simulink model "LAB4_Quanser"  (R2021b)
settings: Solver=VariableStepAuto  StartTime=0.0  StopTime=100  FixedStep=Ts  RelTol=1e-3
InitFcn:
  | Ts=1e-3;
  | Ra = 2.6+2;
  | Ka = 1/Ra;
  | Ta = 500e-6;
  | Tfi = 1e-3;
  | Tsum = 2e-3;
  | KR =1/(2*Ka)*Tfi/Tsum;
  | P = KR;
  | I = KR/Ta;
  | Tfb = 10e-3;
undefined symbols (not defined in the file): Model_626, Sensoray
libraries: sldrtlib x3, simulink x1
settings Model: SimulationMode=external  ExtModeTrigDuration=10001  Creator=Melab1Guest  LastModifiedBy=Marko
settings SolverCC: AlgebraicLoopSolver=TrustRegion
settings SFSimCC: CustomCodeUndefinedFunction=UseInterfaceOnly
settings RTWCC: Description=Simulink Desktop Real-Time  SystemTargetFile=sldrt.tlc  TemplateMakefile=sldrt.tmf  RTWCompilerOptimization=on
settings CodeAppCC: MaxIdLength=95
settings SimulinkDesktopRealTimeCC: TargetPreCompLibLocation=C:\Program Files\MATLAB\R2021b\toolbox\sldrt\lib\win64

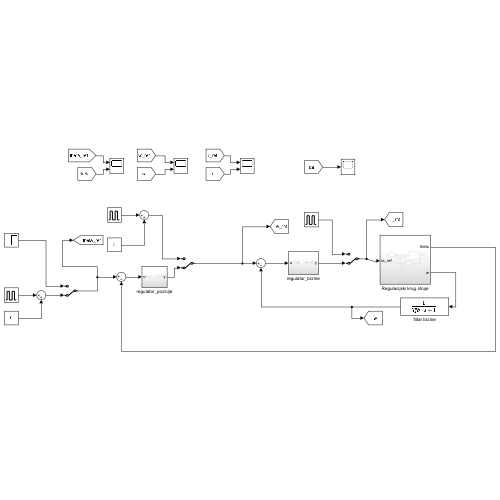
[thumbnail: Simulink's stored preview of the top-level diagram]
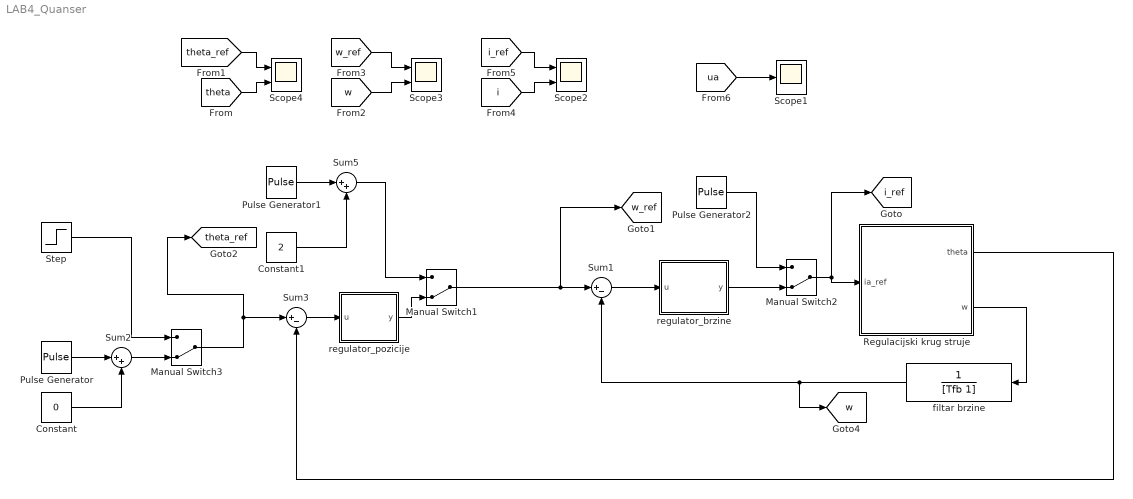
== system LAB4_Quanser ==
  Constant : Constant  Value=0
  Constant1 : Constant  Value=2
  Manual Switch1 : ManualSwitch  CurrentSetting=0
  Manual Switch2 : ManualSwitch  CurrentSetting=0
  Manual Switch3 : ManualSwitch  CurrentSetting=0
  Pulse Generator : DiscretePulseGenerator  PulseType=Time based  Period=10  PulseWidth=50
  Pulse Generator1 : DiscretePulseGenerator  PulseType=Time based  Period=5  PulseWidth=50
  Pulse Generator2 : DiscretePulseGenerator  PulseType=Time based  Amplitude=0.2  Period=3  PulseWidth=50
  Regulacijski krug struje : Subsystem
  Scope1 : Scope
  Scope2 : Scope  NumInputPorts=2
  Scope3 : Scope  NumInputPorts=2
  Scope4 : Scope  NumInputPorts=2
  Step : Step  SampleTime=0
  Sum1 : Sum  Inputs=|+-
  Sum2 : Sum  Inputs=|++
  Sum3 : Sum  Inputs=|+-
  Sum5 : Sum  Inputs=|++
  filtar brzine : TransferFcn  Denominator=[Tfb 1]
  regulator_brzine : Subsystem
  regulator_pozicije : Subsystem
  tag scope: i_ref=global, theta_ref=global, w=global, w_ref=global
  wires:
  Pulse Generator/1 -> Sum2/1
  Constant/1 -> Sum2/2
  Pulse Generator1/1 -> Sum5/1
  Constant1/1 -> Sum5/2
  Sum5/1 -> Manual Switch1/1
  Regulacijski krug struje/1(theta) -> Sum3/2
  Regulacijski krug struje/2(w) -> filtar brzine/1
  Manual Switch2/1 -> [i_ref], Regulacijski krug struje/1(ia_ref)
  Manual Switch3/1 -> Sum3/1, [theta_ref]
  Sum2/1 -> Manual Switch3/2
  Step/1 -> Manual Switch3/1
  filtar brzine/1 -> [w], Sum1/2
  [w_ref] -> Scope3/1
  [w] -> Scope3/2
  [theta] -> Scope4/2
  [theta_ref] -> Scope4/1
  [i_ref] -> Scope2/1
  [i] -> Scope2/2
  Sum3/1 -> regulator_pozicije/1(u)
  regulator_pozicije/1(y) -> Manual Switch1/2
  Sum1/1 -> regulator_brzine/1(u)
  regulator_brzine/1(y) -> Manual Switch2/2
  Pulse Generator2/1 -> Manual Switch2/1
  [ua] -> Scope1/1
  Manual Switch1/1 -> [w_ref], Sum1/1

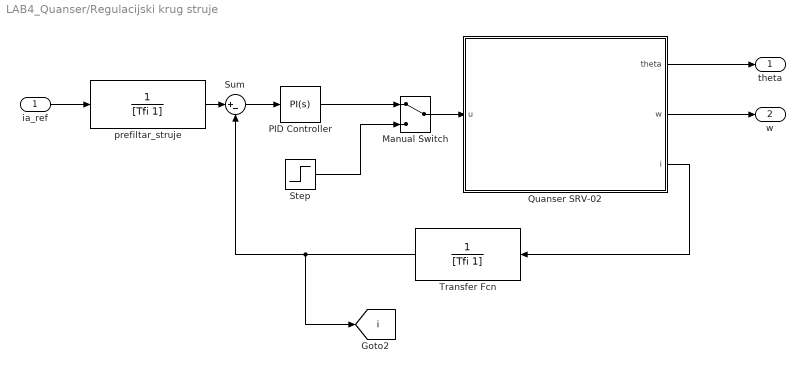
== system LAB4_Quanser/Regulacijski krug struje ==
  ia_ref : Inport
  Manual Switch : ManualSwitch
  PID Controller : simulink/Continuous/PID Controller  Controller=PI  Form=Parallel  TimeDomain=Continuous-time  SampleTime=-1  IntegratorMethod=Forward Euler  FilterMethod=Forward Euler  ControllerParametersSource=internal  P=P  I=I  D=0  UseFilter=on  N=100  TunerSelectOption=Transfer Function Based (PID Tuner App)  InitialConditionSource=internal  InitialConditionForIntegrator=0  InitialConditionForFilter=0  DifferentiatorICPrevScaledInput=0  ExternalReset=none  TrackingMode=off  Kt=1  LimitOutput=on  UpperSaturationLimit=6  LowerSaturationLimit=-6  LinearizeAsGain=on  AntiWindupMode=clamping  Kb=1  POutMin=[]  POutMax=[]  IOutMin=[]  IOutMax=[]  DOutMin=[]  DOutMax=[]  NOutMin=[]  NOutMax=[]  SumOutMin=[]  SumOutMax=[]  SaturationOutMin=[]  SaturationOutMax=[]  PParamMin=[]  PParamMax=[]  IParamMin=[]  IParamMax=[]  DParamMin=[]  DParamMax=[]  NParamMin=[]  NParamMax=[]  KbParamMin=[]  KbParamMax=[]  KtParamMin=[]  KtParamMax=[]  KbOutMin=[]  KbOutMax=[]  KtOutMin=[]  KtOutMax=[]  IntegratorOutMin=[]  IntegratorOutMax=[]  FilterOutMin=[]  FilterOutMax=[]  SumI1OutMin=[]  SumI1OutMax=[]  SumI2OutMin=[]  SumI2OutMax=[]  SumI3OutMin=[]  SumI3OutMax=[]  SumI4OutMin=[]  SumI4OutMax=[]  SumDOutMin=[]  SumDOutMax=[]  DifferentiatorOutMin=[]  DifferentiatorOutMax=[]  FilterDiffOutCoefMin=[]  FilterDiffOutCoefMax=[]  ReciprocalOutMin=[]  ReciprocalOutMax=[]  SumDenOutMin=[]  SumDenOutMax=[]  SumNumOutMin=[]  SumNumOutMax=[]  DivideOutMin=[]  DivideOutMax=[]  IntegratorContinuousStateAttributes=''  IntegratorStateMustResolveToSignalObject=off  IntegratorRTWStateStorageClass=Auto  FilterContinuousStateAttributes=''  FilterStateMustResolveToSignalObject=off  FilterRTWStateStorageClass=Auto  ParallelPVariant=InternalParameters  IdealPVariant=Disabled  IVariant=InternalParameters  DVariant=Disabled  IntegratorVariant=Continuous  SatVariant=Enabled  AWVariant=ContClampingParallel  PCopyVariant=Disabled  TRVariant=Disabled  FdbkBlocksVariant=Forward  IdealPFdbkVariant=Disabled  SatFdbkVariant=Disabled  DerivativeFilterVariant=Disabled  NVariant=Disabled  NCopyVariant=Disabled_SignalSpec  FilterICVariant=Disabled  IntegratorICVariant=InternalICs  ExternalResetVariant=Disabled  TRSumVariant=Passthrough  SumFdbkVariant=Disabled  SumVariant=Sum_PI
  Quanser SRV-02 : Subsystem
  Step : Step  After=6  SampleTime=0
  Sum : Sum  Inputs=|+-
  Transfer Fcn : TransferFcn  Denominator=[Tfi 1]
  prefiltar_struje : TransferFcn  Denominator=[Tfi 1]
  theta : Outport
  w : Outport  Port=2
  tag scope: i=global
  wires:
  prefiltar_struje/1 -> Sum/1
  Sum/1 -> PID Controller/1
  PID Controller/1 -> Manual Switch/1
  Quanser SRV-02/1(theta) -> theta/1
  Manual Switch/1 -> Quanser SRV-02/1(u)
  Step/1 -> Manual Switch/2
  Quanser SRV-02/2(w) -> w/1
  ia_ref/1 -> prefiltar_struje/1
  Transfer Fcn/1 -> [i], Sum/2
  Quanser SRV-02/3(i) -> Transfer Fcn/1

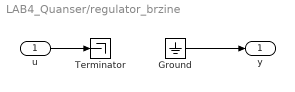
== system LAB4_Quanser/regulator_brzine ==
  u : Inport
  Ground : Ground
  Terminator : Terminator
  y : Outport
  wires:
  u/1 -> Terminator/1
  Ground/1 -> y/1

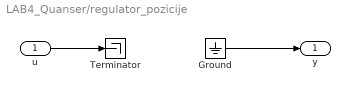
== system LAB4_Quanser/regulator_pozicije ==
  u : Inport
  Ground : Ground
  Terminator : Terminator
  y : Outport
  wires:
  Ground/1 -> y/1
  u/1 -> Terminator/1

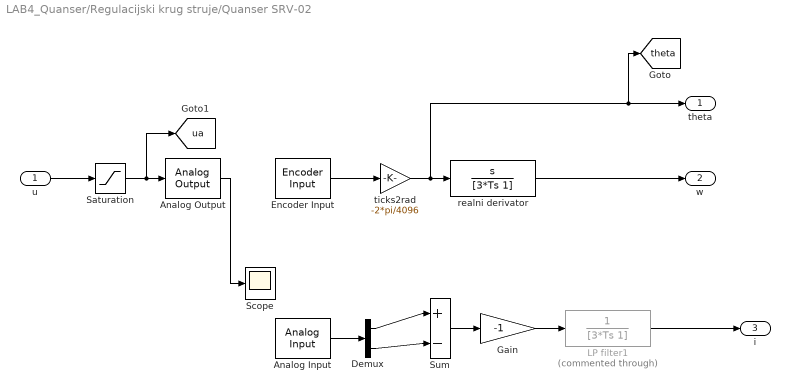
== system LAB4_Quanser/Regulacijski krug struje/Quanser SRV-02 ==
  u : Inport
  Analog Input : sldrtlib/Analog Input  SampleTime=Ts  MaxMissedTicks=100  ShowMissedTicks=off  YieldWhenWaiting=off  DrvName=Sensoray/Model_626  DrvAddress=4294967295  DrvOptions=zeros(1,0)  Channels=[1,2]  RangeMode=1  VoltRange=2  DataType=1
      settings: AttributesFormatString=Sensoray\nModel 626 [auto]
  Analog Output : sldrtlib/Analog Output  SampleTime=Ts  MaxMissedTicks=100  ShowMissedTicks=on  YieldWhenWaiting=off  DrvName=Sensoray/Model_626  DrvAddress=4294967295  DrvOptions=zeros(1,0)  Channels=1  RangeMode=1  VoltRange=1  InitialValue=0  FinalValue=0
      settings: AttributesFormatString=Sensoray\nModel 626 [auto]
  Demux : Demux  Outputs=2
  Encoder Input : sldrtlib/Encoder Input  SampleTime=Ts  MaxMissedTicks=100  ShowMissedTicks=off  YieldWhenWaiting=off  DrvName=Sensoray/Model_626  DrvAddress=4294967295  DrvOptions=zeros(1,0)  Channels=1  QuadMode=3  IndexPulse=2  InputFilter=Inf  DataType=1
      settings: AttributesFormatString=Sensoray\nModel 626 [auto]
  Gain : Gain  Gain=-1
  LP filter1 : TransferFcn  Commented=through  Denominator=[3*Ts 1]
  Saturation : Saturate  UpperLimit=4  LowerLimit=-4
  Scope : Scope
  Sum : Sum  Inputs=|+-
  realni derivator : TransferFcn  Numerator=[1 0]  Denominator=[3*Ts 1]
  ticks2rad : Gain  Gain=-2*pi/4096
  theta : Outport
  w : Outport  Port=2
  i : Outport  Port=3
  tag scope: theta=global, ua=global
  wires:
  Encoder Input/1 -> ticks2rad/1
  Analog Output/1 -> Scope/1
  u/1 -> Saturation/1
  Saturation/1 -> [ua], Analog Output/1
  Analog Input/1 -> Demux/1
  Sum/1 -> Gain/1
  Demux/2 -> Sum/2
  Demux/1 -> Sum/1
  Gain/1 -> LP filter1/1
  LP filter1/1 -> i/1
  realni derivator/1 -> w/1
  ticks2rad/1 -> [theta], theta/1, realni derivator/1
